simulink model "Main_2024_UDP_confirmed_2024a"  (R2024a)
settings: Solver=ode1  StartTime=0.0  StopTime=inf  FixedStep=0.01  RelTol=1e-3  EnableMultiTasking=on
undefined symbols (not defined in the file or in its folder): gray
settings Model: ExplicitPartitioning=on  Creator=최지웅  LastModifiedBy=LG gram 17 - HW dev
settings SolverCC: PositivePriorityOrder=on
settings DebuggingCC: AlgebraicLoopMsg=none
settings HardwareCC: ProdBitPerLong=64  ProdHWDeviceType=Intel->x86-64 (Linux 64)
settings RTWCC: Description=Simulink Desktop Real-Time  SystemTargetFile=sldrt.tlc  TemplateMakefile=sldrt.tmf  RTWCompilerOptimization=on  GPUComputeCapability=3.5
settings CodeAppCC: MaxIdLength=95
settings SimulinkDesktopRealTimeCC: TargetLibSuffix=_sldrt.a  TargetPreCompLibLocation=C:\Program Files\MATLAB\R2024a\toolbox\sldrt\lib\win64

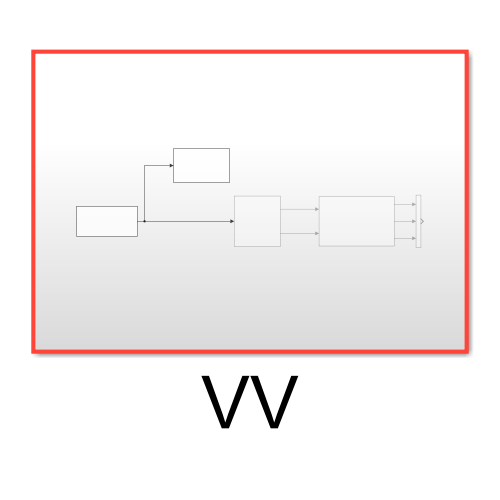
[thumbnail: Simulink's stored preview of the top-level diagram]
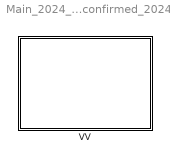
== system Main_2024_UDP_confirmed_2024a ==
  VV : Subsystem

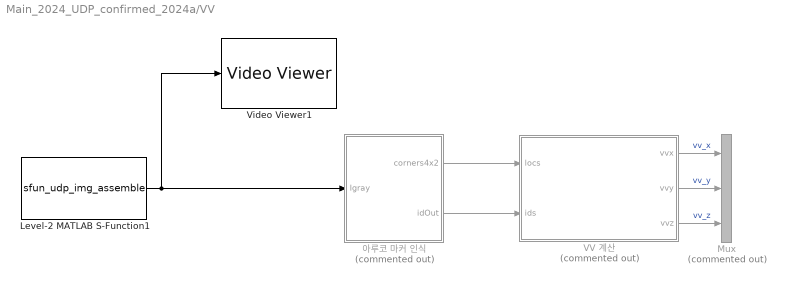
== system Main_2024_UDP_confirmed_2024a/VV ==
  Level-2 MATLAB S-Function1 : M-S-Function  FunctionName=sfun_udp_img_assemble  Parameters=5006, [480 640], 8192, 0.1
  Mux : Mux  Commented=on  Inputs=3
  VV 계산 : MATLAB Function  Commented=on  TreatAsAtomicUnit=on
  Video Viewer1 : VideoViewer  colormapValue=gray(256)  FigPos=[248.428571428571 730 652 453.714285714286]
  아루코 마커 인식 : MATLAB Function  Commented=on  TreatAsAtomicUnit=on
  wires:
  VV 계산/3(vvz) -> Mux/3  "vv_z"
  아루코 마커 인식/2(idOut) -> VV 계산/2(ids)
  VV 계산/1(vvx) -> Mux/1  "vv_x"
  VV 계산/2(vvy) -> Mux/2  "vv_y"
  아루코 마커 인식/1(corners4x2) -> VV 계산/1(locs)
  Level-2 MATLAB S-Function1/1 -> Video Viewer1/1, 아루코 마커 인식/1(Igray)

== matlab function Main_2024_UDP_confirmed_2024a/VV/아루코 마커 인식 ==
  data: Igray input; corners4x2 output; idOut output
function [corners4x2, idOut] = fcn(Igray)
% 한 개의 ArUco 마커만 검출
%   Igray      : uint8 [H×W] 그레이스케일 이미지
%   corners4x2 : double [4×2] 검출된 마커의 네 꼭짓점 좌표
%   idOut      : uint16     검출된 마커의 ID (없으면 0)
%
% R2024a 이상 환경에서  동작


    %#codegen
    coder.extrinsic('readArucoMarker');

    %출력 초기화 (고정 크기, 고정 타입) —%
    corners4x2 = zeros(4,2);   % [4×2] double
    idOut      = uint16(0);    % 스칼라 uint16
    if isempty(Igray)
        return;
    end

    %ArUco 검출 (시뮬레이션에서만 실행) —%
    [idsDetected, locsDetected] = readArucoMarker(Igray, "DICT_6X6_250");
    if isempty(idsDetected)
        return;
    end

    %첫 번째 마커 정보만 사용 —%
    idTemp = idsDetected(1);         % extrinsic 호출 결과(double)
    idOut  = uint16(idTemp);

    corners4x2(1,1) = locsDetected(1,1,1);
    corners4x2(1,2) = locsDetected(1,2,1);
    corners4x2(2,1) = locsDetected(2,1,1);
    corners4x2(2,2) = locsDetected(2,2,1);
    corners4x2(3,1) = locsDetected(3,1,1);
    corners4x2(3,2) = locsDetected(3,2,1);
    corners4x2(4,1) = locsDetected(4,1,1);
    corners4x2(4,2) = locsDetected(4,2,1);
end

== matlab function Main_2024_UDP_confirmed_2024a/VV/VV 계산 ==
  data: locs input; vvx output; ids input; vvy output; vvz output
function [vvx, vvy, vvz] = tiltVV(locs, ids)
% locs:    [4×2×N] double - 각 마커의 네 꼭짓점 좌표 (x,y)
% ids:     [N×1] uint16  - 각 마커 ID
% vvx, vvy, vvz: 실시간으로 계산된 VV 벡터 성분

    %% 1) 만약 마커가 하나도 검출되지 않았다면 0 출력
    if isempty(ids)
        vvx = 0;
        vvy = 0;
        vvz = 0;
        return;
    end

    %% 2) 첫 번째 마커만 사용 (추가 검출 마커는 무시)
    % locs(:,:,1) -> [4×2] 배열: 
    %   row 1: top-left  (x1, y1)
    %   row 2: top-right (x2, y2)
    %   row 3: bot-right (x3, y3)
    %   row 4: bot-left  (x4, y4)
    corners = locs(:,:,1);   % [4×2]
    % Top-left = corners(1,:), Top-right = corners(2,:)
    x1 = corners(1,1);  y1 = corners(1,2);
    x2 = corners(2,1);  y2 = corners(2,2);

    %% 3) dx, dy 계산 (영상좌표계 기준 → 화면상의 x,y 차이)
    dx = double(x2 - x1);
    dy = double(y2 - y1);

    %% 4) raw_angle 계산 (deg 단위), arctan2(dy, dx) → 라디안 → 도
    raw_rad  = atan2(dy, dx);               % -pi ~ +pi (rad)
    raw_deg  = rad2deg(raw_rad);            % -180 ~ +180 (deg)
    raw_angle = mod(raw_deg + 360, 360);    % 0 ~ 360

    %% 5) tilt 계산 (0~180 범위로 매핑)
    % tilt = ( 90 – raw_angle ) mod 360, 
    % 만약 결과 > 180 이면 360 – 결과
    temp = mod(90 - raw_angle + 360, 360);  
    if temp > 180
        tilt = 360 - temp;
    else
        tilt = temp;
    end

    %% 6) 중력 가속도 (m/s^2)
    g = 9.81;

    %% 7) tilt → 라디안
    theta = deg2rad(tilt);

    %% 8) VV 벡터 성분 계산
    vvx = g * cos(theta);   % 영상 기준 x축 방향 성분
    vvy = g * sin(theta);   % 영상 기준 y축 방향 성분
    vvz = 0;                % 2D 영상이므로 z 성분은 0으로 고정
end
